simulink subsystem "ProcNav"  (R2024a)
settings: Solver=VariableStepAuto  StartTime=0.0  StopTime=10.0  RelTol=1e-3
undefined symbols (not defined in the file): DiscIntNeverNeededParam, physics, simulation, simulink
libraries: aerolibutil x7, sharedtransform x1, simulink x1, sharedTrackingLibrary x1
settings Model: Creator=Lamarre  LastModifiedBy=sonia2
settings SolverCC: AlgebraicLoopSolver=TrustRegion
settings DebuggingCC: UnconnectedInputMsg=warning  UnconnectedOutputMsg=warning  UnconnectedLineMsg=warning
settings ModelReferenceCC: EnableRefExpFcnMdlSchedulingChecks=on
settings RTWCC: GPUComputeCapability=3.5  DLArmComputeVersion=19.05

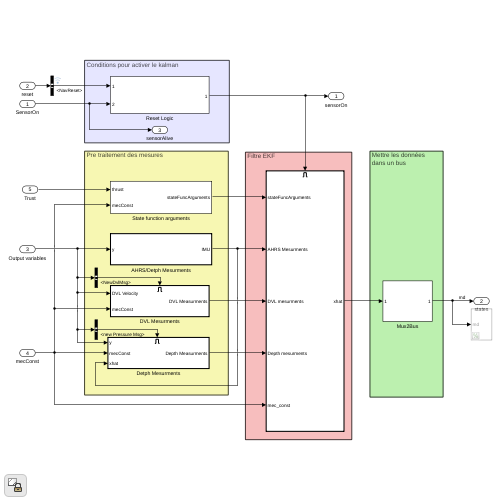
[thumbnail: Simulink's stored preview of the top-level diagram]
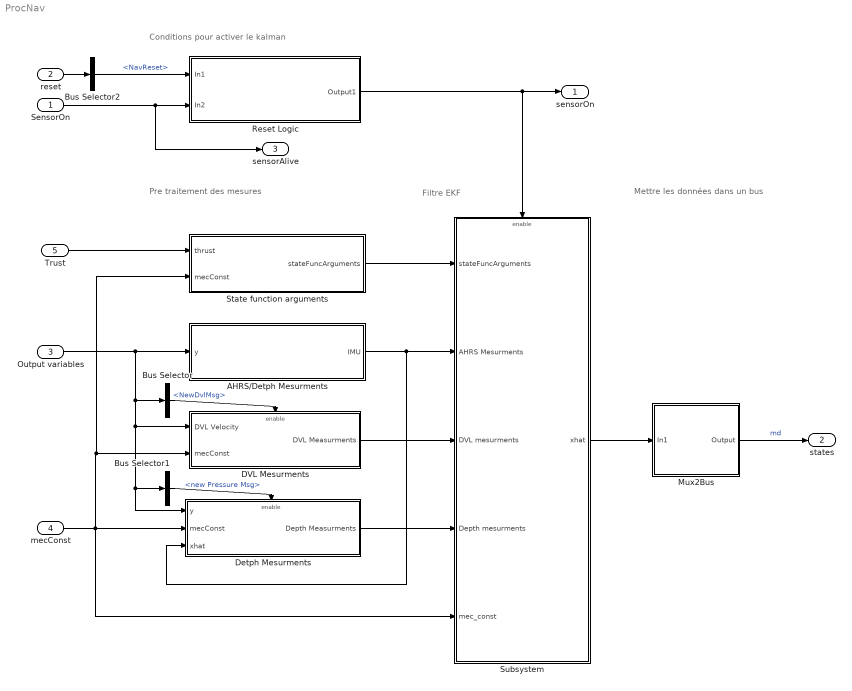
== system ProcNav ==
  note: Conditions pour activer le kalman
  note: Filtre EKF
  note: Pre traitement des mesures
  note: Mettre les données
      | dans un bus
  SensorOn : Inport
  reset : Inport  Port=2
  Output variables : Inport  Port=3
  mecConst : Inport  Port=4
  Trust : Inport  Port=5
  AHRS/Detph Mesurments : Subsystem  TreatAsAtomicUnit=on  SystemSampleTime=simulink.procNav.sampletime
  Bus Selector : BusSelector  OutputSignals=NewDvlMsg
  Bus Selector1 : BusSelector  OutputSignals=new Pressure Msg
  Bus Selector2 : BusSelector  OutputSignals=NavReset
  DVL Mesurments : Subsystem
  Detph Mesurments : Subsystem  TreatAsAtomicUnit=on  SystemSampleTime=simulink.procNav.sampletime
  Mux2Bus : Subsystem
  Reset Logic : Subsystem
  State function arguments : Subsystem
  Subsystem : Subsystem
  sensorOn : Outport
  states : Outport  Port=2
  sensorAlive : Outport  Port=3
  wires:
  AHRS/Detph Mesurments/1(IMU) -> Subsystem/2(AHRS Mesurments), Detph Mesurments/3(xhat)
  DVL Mesurments/1(DVL Measurments) -> Subsystem/3(DVL mesurments)
  Subsystem/1(xhat) -> Mux2Bus/1(In1)
  Output variables/1 -> AHRS/Detph Mesurments/1(y), Bus Selector/1, DVL Mesurments/1(DVL Velocity), Detph Mesurments/1(y), Bus Selector1/1
  Trust/1 -> State function arguments/1("thrust ")
  reset/1 -> Bus Selector2/1
  SensorOn/1 -> Reset Logic/2(In2), sensorAlive/1
  Mux2Bus/1(Output) -> states/1  "md"
  Bus Selector/1 -> DVL Mesurments/Enable  "<NewDvlMsg>"
  Reset Logic/1(Output1) -> Subsystem/Enable, sensorOn/1
  Detph Mesurments/1(Depth Measurments) -> Subsystem/4(Depth mesurments)
  Bus Selector1/1 -> Detph Mesurments/Enable  "<new Pressure Msg>"
  Bus Selector2/1 -> Reset Logic/1(In1)  "<NavReset>"
  mecConst/1 -> Detph Mesurments/2(mecConst), DVL Mesurments/2(mecConst), State function arguments/2(mecConst), Subsystem/5(mec_const)
  State function arguments/1(stateFuncArguments) -> Subsystem/1(stateFuncArguments)

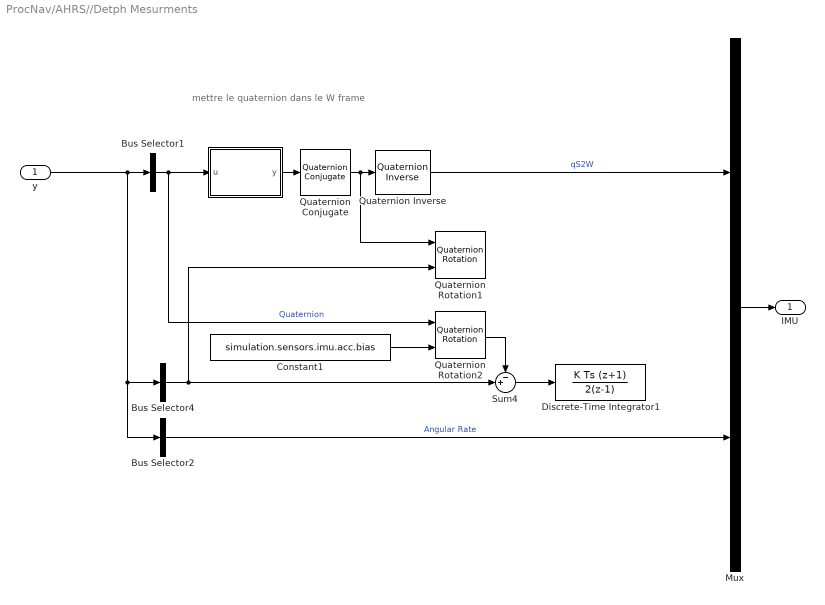
== system ProcNav/AHRS//Detph Mesurments ==
  note: mettre le quaternion dans
      | le W frame
  y : Inport
  " " : MATLAB Function  TreatAsAtomicUnit=on
  Bus Selector1 : BusSelector  OutputSignals=Quaternion  OutputAsBus=on
  Bus Selector2 : BusSelector  OutputSignals=Angular Rate  OutputAsBus=on
  Bus Selector4 : BusSelector  OutputSignals=Linear Acc  OutputAsBus=on
  Constant1 : Constant  Value=simulation.sensors.imu.acc.bias
  Discrete-Time Integrator1 : DiscreteIntegrator  IntegratorMethod=Integration: Trapezoidal  SampleTime=-1  ICPrevOutput=DiscIntNeverNeededParam  ICPrevScaledInput=DiscIntNeverNeededParam
  Mux : Mux  Inputs=2
  Quaternion Conjugate : aerolibutil/Quaternion Conjugate
  Quaternion Inverse : aerolibutil/Quaternion Inverse
  Quaternion Rotation1 : aerolibutil/Quaternion Rotation
  Quaternion Rotation2 : aerolibutil/Quaternion Rotation
  Sum4 : Sum  Inputs=-+|
  IMU : Outport
  wires:
  " "/1(y) -> Quaternion Conjugate/1
  Sum4/1 -> Discrete-Time Integrator1/1
  Quaternion Rotation2/1 -> Sum4/1
  Constant1/1 -> Quaternion Rotation2/2
  Bus Selector4/1 -> Quaternion Rotation1/2, Sum4/2
  Quaternion Conjugate/1 -> Quaternion Rotation1/1, Quaternion Inverse/1
  Mux/1 -> IMU/1
  Bus Selector2/1 -> Mux/2  "Angular Rate"
  Quaternion Inverse/1 -> Mux/1  "qS2W"
  Bus Selector1/1 -> Quaternion Rotation2/1, " "/1(u)  "Quaternion"
  y/1 -> Bus Selector1/1, Bus Selector4/1, Bus Selector2/1

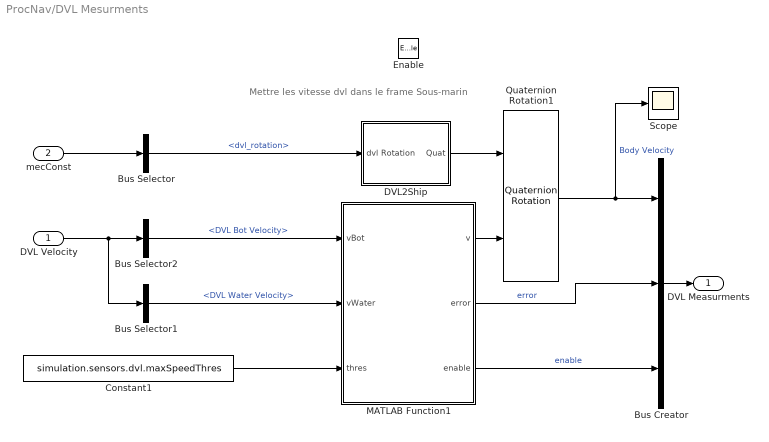
== system ProcNav/DVL Mesurments ==
  note: Mettre les vitesse dvl dans le frame Sous-marin
  DVL Velocity : Inport
  mecConst : Inport  Port=2
  Enable : EnablePort
  Bus Creator : BusCreator  Inputs=3
  Bus Selector : BusSelector  OutputSignals=dvl_rotation
  Bus Selector1 : BusSelector  OutputSignals=DVL Water Velocity
  Bus Selector2 : BusSelector  OutputSignals=DVL Bot Velocity
  Constant1 : Constant  Value=simulation.sensors.dvl.maxSpeedThres
  DVL2Ship : Subsystem
  MATLAB Function1 : MATLAB Function  TreatAsAtomicUnit=on
  Quaternion Rotation1 : aerolibutil/Quaternion Rotation
  Scope : Scope
  DVL Measurments : Outport
  wires:
  Bus Selector/1 -> DVL2Ship/1(dvl Rotation)  "<dvl_rotation>"
  mecConst/1 -> Bus Selector/1
  Bus Creator/1 -> DVL Measurments/1
  MATLAB Function1/2(error) -> Bus Creator/2  "error"
  MATLAB Function1/3(enable) -> Bus Creator/3  "enable"
  Quaternion Rotation1/1 -> Bus Creator/1, Scope/1  "Body Velocity"
  Bus Selector1/1 -> MATLAB Function1/2(vWater)  "<DVL Water Velocity>"
  Bus Selector2/1 -> MATLAB Function1/1(vBot)  "<DVL Bot Velocity>"
  DVL Velocity/1 -> Bus Selector2/1, Bus Selector1/1
  MATLAB Function1/1(v) -> Quaternion Rotation1/2
  Constant1/1 -> MATLAB Function1/3(thres)
  DVL2Ship/1(Quat) -> Quaternion Rotation1/1

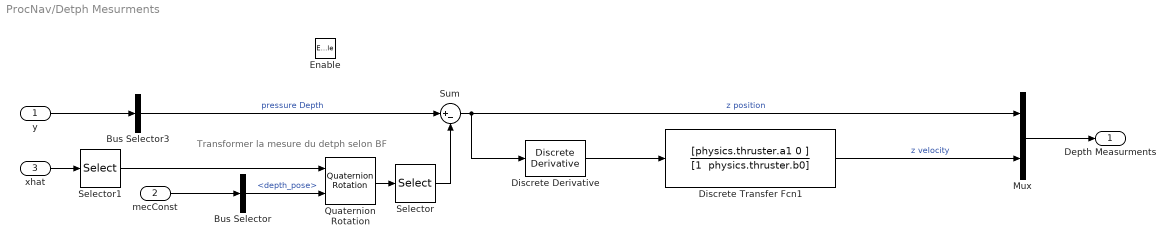
== system ProcNav/Detph Mesurments ==
  note: Transformer la mesure du detph selon BF
  y : Inport
  mecConst : Inport  Port=2
  xhat : Inport  Port=3
  Enable : EnablePort
  Bus Selector : BusSelector  OutputSignals=depth_pose
  Bus Selector3 : BusSelector  OutputSignals=Pressure Depth  OutputAsBus=on
  Discrete Transfer Fcn1 : DiscreteTransferFcn  Numerator=[physics.thruster.a1 0 ]  Denominator="[1  physics.thruster.b0]"  SampleTime=1/50
  Discrete Derivative : simulink/Discrete/Discrete Derivative  gainval=1.0  ICPrevScaledInput=0.0  OutMin=[]  OutMax=[]  OutDataType=fixdt(1, 16)  OutScaling=2^-10  DoSatur=off
  Mux : Mux  Inputs=2
  Quaternion Rotation : aerolibutil/Quaternion Rotation
  Selector : Selector  InputPortWidth=3  IndexOptions=Index vector (dialog)  Indices=[3]  OutputSizes=1
  Selector1 : Selector  InputPortWidth=7  IndexOptions=Index vector (dialog)  Indices=[1:4]  OutputSizes=1
  Sum : Sum  Inputs=|+-
  Depth Measurments : Outport
  wires:
  mecConst/1 -> Bus Selector/1
  Selector1/1 -> Quaternion Rotation/1
  xhat/1 -> Selector1/1
  y/1 -> Bus Selector3/1
  Discrete Transfer Fcn1/1 -> Mux/2  "z velocity"
  Discrete Derivative/1 -> Discrete Transfer Fcn1/1
  Sum/1 -> Discrete Derivative/1, Mux/1  "z position"
  Quaternion Rotation/1 -> Selector/1
  Selector/1 -> Sum/2
  Bus Selector/1 -> Quaternion Rotation/2  "<depth_pose>"
  Bus Selector3/1 -> Sum/1  "pressure Depth"
  Mux/1 -> Depth Measurments/1

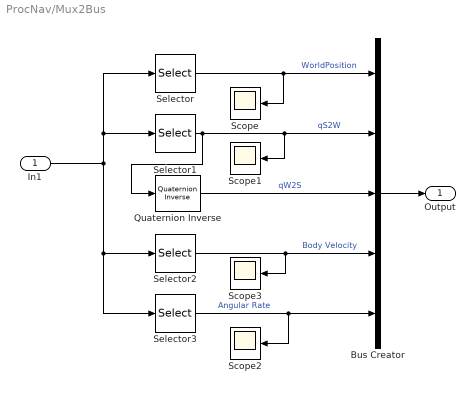
== system ProcNav/Mux2Bus ==
  In1 : Inport
  Bus Creator : BusCreator  Inputs=5
  Quaternion Inverse : aerolibutil/Quaternion Inverse
  Scope{,1..3} (4 alike) : Scope
  Selector : Selector  InputPortWidth=13  IndexOptions=Index vector (dialog)  Indices=[1:3]  OutputSizes=1
  Selector1 : Selector  InputPortWidth=13  IndexOptions=Index vector (dialog)  Indices=[4:7]  OutputSizes=1
  Selector2 : Selector  InputPortWidth=13  IndexOptions=Index vector (dialog)  Indices=[8:10]  OutputSizes=1
  Selector3 : Selector  InputPortWidth=13  IndexOptions=Index vector (dialog)  Indices=[11:13]  OutputSizes=1
  Output : Outport
  wires:
  Quaternion Inverse/1 -> Bus Creator/3  "qW2S"
  Selector2/1 -> Scope3/1, Bus Creator/4  "Body Velocity"
  Selector3/1 -> Scope2/1, Bus Creator/5  "Angular Rate"
  In1/1 -> Selector/1, Selector1/1, Selector2/1, Selector3/1
  Selector/1 -> Bus Creator/1, Scope/1  "WorldPosition"
  Selector1/1 -> Bus Creator/2, Scope1/1, Quaternion Inverse/1  "qS2W"
  Bus Creator/1 -> Output/1

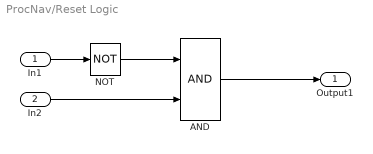
== system ProcNav/Reset Logic ==
  In1 : Inport
  In2 : Inport  Port=2
  AND : Logic  AllPortsSameDT=off  OutDataTypeStr=boolean
  NOT : Logic  Operator=NOT  AllPortsSameDT=off  OutDataTypeStr=boolean
  Output1 : Outport
  wires:
  AND/1 -> Output1/1
  In1/1 -> NOT/1
  NOT/1 -> AND/1
  In2/1 -> AND/2

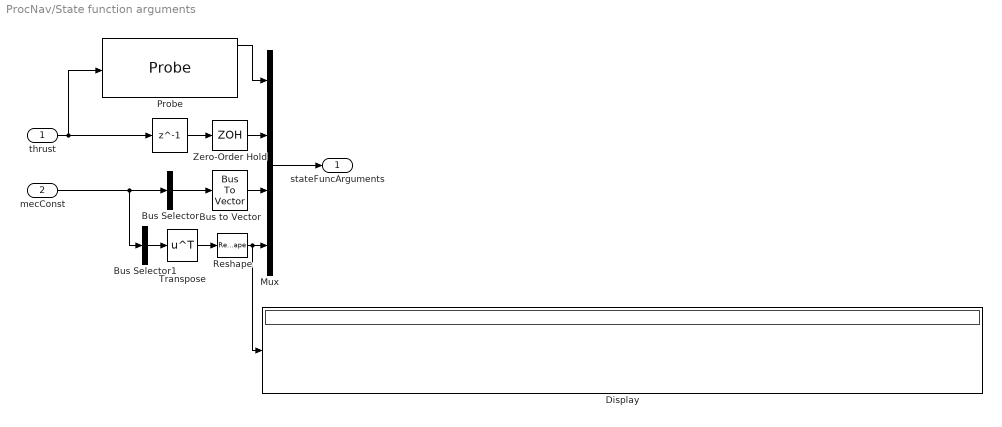
== system ProcNav/State function arguments ==
  "thrust " : Inport
  mecConst : Inport  Port=2
  " " : Delay  DelayLength=1  InitialCondition=[0,0,0,0,0,0,0,0]
  Bus Selector : BusSelector  OutputSignals=mass,volume,sub_height,I,rg,rb,cdl,cdq,added_mass,rho,g  OutputAsBus=on
  Bus Selector1 : BusSelector  OutputSignals=thrusters  OutputAsBus=on
  Bus to Vector : BusToVector
  Display : Display
  Mux : Mux
  Probe : Probe  ProbeSignalDimensions=on
  Reshape : Reshape
  Transpose : Math  Operator=transpose
  Zero-Order Hold : ZeroOrderHold  SampleTime=simulink.procNav.sampletime
  stateFuncArguments : Outport
  wires:
  Probe/1 -> Mux/1
  Reshape/1 -> Mux/4, Display/1
  Bus Selector1/1 -> Transpose/1
  Transpose/1 -> Reshape/1
  Mux/1 -> stateFuncArguments/1
  Bus to Vector/1 -> Mux/3
  Zero-Order Hold/1 -> Mux/2
  Bus Selector/1 -> Bus to Vector/1
  mecConst/1 -> Bus Selector/1, Bus Selector1/1
  " "/1 -> Zero-Order Hold/1
  "thrust "/1 -> Probe/1, " "/1

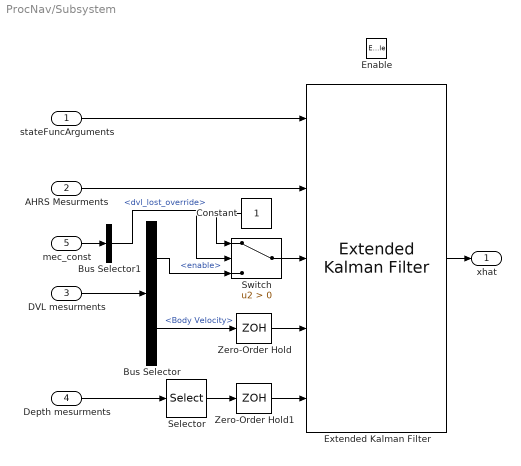
== system ProcNav/Subsystem ==
  stateFuncArguments : Inport
  AHRS Mesurments : Inport  Port=2
  DVL mesurments : Inport  Port=3
  Depth mesurments : Inport  Port=4
  mec_const : Inport  Port=5
  Enable : EnablePort  StatesWhenEnabling=reset
  Bus Selector : BusSelector  OutputSignals=enable,Body Velocity
  Bus Selector1 : BusSelector  OutputSignals=dvl_lost_override
  Constant : Constant
  Extended Kalman Filter : sharedTrackingLibrary/Extended Kalman Filter  StateTransitionFcn=EkfNavStatesEq  HasStateTransitionJacobianFcn=off  StateTransitionJacobianFcn=EkfNavJacobian  HasAdditiveProcessNoise=Additive  ProcessNoise=kalman.Cx  HasTimeVaryingProcessNoise=off  HasStateTransitionFcnExtraArgument=1  InitialState=kalman.Xi  InitialStateCovariance=kalman.Ci  MeasurementFcn1=EkfNavAhrs  HasMeasurementJacobianFcn1=off  MeasurementJacobianFcn1=EkfJacobianNavAhrsDepth  HasMeasurementEnablePort1=off  HasAdditiveMeasurementNoise1=Additive  MeasurementNoise1=kalman.Cimu  HasTimeVaryingMeasurementNoise1=off  HasMeasurementFcnExtraArgument1=0  HasMeasurementWrapping1=off  MeasurementFcn2=EkfNavDvl  HasMeasurementJacobianFcn2=off  MeasurementJacobianFcn2=EkfJacobianNavDvl  HasMeasurementEnablePort2=on  HasAdditiveMeasurementNoise2=Additive  MeasurementNoise2=kalman.Cdvl  HasTimeVaryingMeasurementNoise2=off  HasMeasurementFcnExtraArgument2=0  HasMeasurementWrapping2=off  MeasurementFcn3=EkfNavDepth  HasMeasurementJacobianFcn3=off  HasMeasurementEnablePort3=off  HasAdditiveMeasurementNoise3=Additive  MeasurementNoise3=kalman.Cdepth  HasTimeVaryingMeasurementNoise3=off  HasMeasurementFcnExtraArgument3=0  HasMeasurementWrapping3=off  MeasurementFcn4=myMeasurementFcn  HasMeasurementJacobianFcn4=off  HasMeasurementEnablePort4=off  HasAdditiveMeasurementNoise4=Additive  MeasurementNoise4=1  HasTimeVaryingMeasurementNoise4=off  HasMeasurementFcnExtraArgument4=0  HasMeasurementWrapping4=off  MeasurementFcn5=myMeasurementFcn  HasMeasurementJacobianFcn5=off  HasMeasurementEnablePort5=off  HasAdditiveMeasurementNoise5=Additive  MeasurementNoise5=1  HasTimeVaryingMeasurementNoise5=off  HasMeasurementFcnExtraArgument5=0  HasMeasurementWrapping5=off  EnableMultirate=on  StateTransitionFcnSampleTime=simulink.procNav.sampletime  MeasurementFcn1SampleTime=simulink.procNav.imuDepth.sampletime  MeasurementFcn2SampleTime=simulink.procNav.dvl.sampletime  MeasurementFcn3SampleTime=simulation.sensors.depth.sampletime  MeasurementFcn4SampleTime=1  MeasurementFcn5SampleTime=1  UseCurrentEstimator=on  OutputStateCovariance=off  DataType=double  SampleTime=simulink.procNav.sampletime  NumberOfMeasurements=3
  Selector : Selector  InputPortWidth=2  IndexOptions=Index vector (dialog)  Indices=[1]  OutputSizes=1
  Switch : Switch  Criteria=u2 > Threshold  SaturateOnIntegerOverflow=off  InputSameDT=off
  Zero-Order Hold : ZeroOrderHold  SampleTime=simulink.procNav.dvl.sampletime
  Zero-Order Hold1 : ZeroOrderHold  SampleTime=simulation.sensors.depth.sampletime
  xhat : Outport
  wires:
  Switch/1 -> Extended Kalman Filter/3
  Constant/1 -> Switch/1
  Bus Selector1/1 -> Switch/2  "<dvl_lost_override>"
  mec_const/1 -> Bus Selector1/1
  Bus Selector/1 -> Switch/3  "<enable>"
  Selector/1 -> Zero-Order Hold1/1
  Zero-Order Hold1/1 -> Extended Kalman Filter/5
  Bus Selector/2 -> Zero-Order Hold/1  "<Body Velocity>"
  Depth mesurments/1 -> Selector/1
  DVL mesurments/1 -> Bus Selector/1
  Zero-Order Hold/1 -> Extended Kalman Filter/4
  AHRS Mesurments/1 -> Extended Kalman Filter/2
  stateFuncArguments/1 -> Extended Kalman Filter/1
  Extended Kalman Filter/1 -> xhat/1

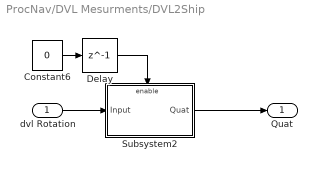
== system ProcNav/DVL Mesurments/DVL2Ship ==
  dvl Rotation : Inport
  Constant6 : Constant  Value=0
  Delay : Delay  DelayLength=1  InitialCondition=1
  Subsystem2 : Subsystem
  Quat : Outport
  wires:
  dvl Rotation/1 -> Subsystem2/1(Input)
  Delay/1 -> Subsystem2/Enable
  Constant6/1 -> Delay/1
  Subsystem2/1(Quat) -> Quat/1

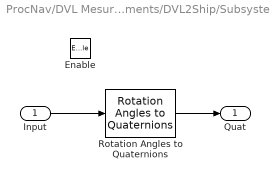
== system ProcNav/DVL Mesurments/DVL2Ship/Subsystem2 ==
  Input : Inport
  Enable : EnablePort
  Rotation Angles to Quaternions : sharedtransform/Rotation Angles to Quaternions  rotationOrder=XYZ  aMode=aMode
  Quat : Outport
  wires:
  Rotation Angles to Quaternions/1 -> Quat/1
  Input/1 -> Rotation Angles to Quaternions/1

== matlab function ProcNav/DVL Mesurments/MATLAB Function1 ==
  data: vBot input; vWater input; v output; error output; thres input; enable output
function [v, error, enable] = DVLManager(vBot,vWater,thres)

    if max(abs(vBot(1:3)))< thres
        %retouner les vitesse du bottom tracking (normal)
        v = vBot(1:3);
        enable = 1;
        error = ones(1,3) * vBot(4);
    elseif max(abs(vWater))< thres
        % retouner les vitesse du water profiling si bottom tracking fail
        v = vWater(1:3);
        enable = 0;
        error = ones(1,3) * vWater(4);
    else
        % Désactiver le dvl si mauvais data
        v = zeros(3,1);
        v(3)= 0;% patch(2);
        enable = 0;
        error = ones(1,3) * vBot(4);
    end
end

== matlab function ProcNav/AHRS//Detph Mesurments/  ==
  data: u input size=4; y output size=4
function y = Normalize(u)
%Normailse le quaternions pour éviter la distortions crée par l'erreur de
% de l'intégration.
d=norm(u);
n=u/d;
if isnan(n)
    y=[1;0;0;0];
else
    y = n;
end
